simulink model "untitled"  (R2024b)
settings: Solver=FixedStepAuto  StartTime=0.0  StopTime=100  FixedStep=0.001  RelTol=1e-3  EnableMultiTasking=on
libraries: arduinolib x4
settings Model: ExtModeTrigDuration=2  Creator=abdal  LastModifiedBy=abdal
settings SolverCC: AutoInsertRateTranBlk=on
settings OptimizationCC: EnhancedBackFolding=on  PassReuseOutputArgsAs=Individual arguments  ZeroExternalMemoryAtStartup=off  ZeroInternalMemoryAtStartup=off  MaxStackSize=64  OptimizeBlockOrder=speed  DifferentSizesBufferReuse=on  OptimizationCustomize=off  EfficientTunableParamExpr=on
settings DebuggingCC: ParameterTunabilityLossMsg=error
settings HardwareCC: ProdBitPerInt=16  ProdBitPerPointer=16  ProdBitPerSizeT=16  ProdBitPerPtrDiffT=16  ProdLargestAtomicFloat=None  ProdWordSize=8  ProdHWDeviceType=Atmel->AVR
settings SFSimCC: MATLABDynamicMemAlloc=off
settings RTWCC: Description=Embedded Coder  SystemTargetFile=ert.tlc  HardwareBoard=Arduino Uno  TemplateMakefile=ert_default_tmf  Toolchain=Arduino AVR  BuildConfiguration=Faster Runs
settings CodeAppCC: ForceParamTrailComments=on  IgnoreCustomStorageClasses=off  OperatorAnnotations=on  SimulinkDataObjDesc=on  SFDataObjDesc=on  InsertBlockDesc=on
settings ERTTargetCC: SupportContinuousTime=on  SupportVariableSizeSignals=on  ExtModeTransport=3  ExtModeStaticAlloc=on  ExtModeAutomaticAllocSize=off  ExtModeStaticAllocSize=250  ExtModeMexFile=ext_xcp  ExtModeIntrfLevel=Level2 - Open  InlinedParameterPlacement=Hierarchical

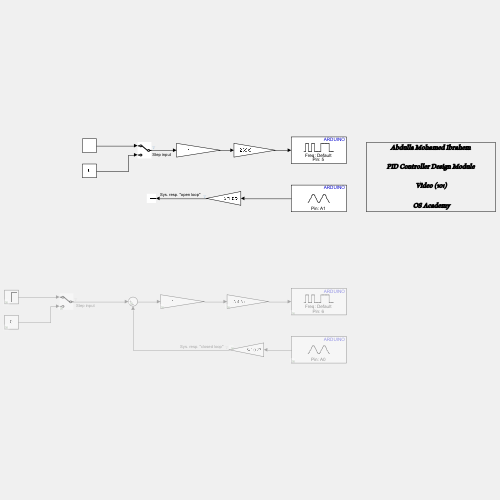
[thumbnail: Simulink's stored preview of the top-level diagram]
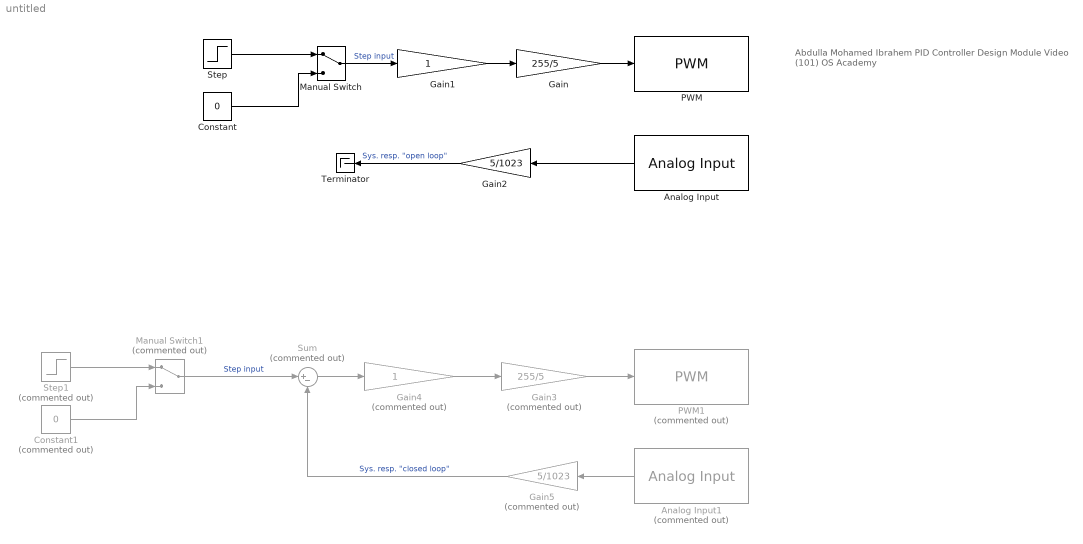
== system untitled ==
  note: Abdulla Mohamed Ibrahem
      | PID Controller Design Module
      | Video (101)
      | OS Academy
  Analog Input : arduinolib/Analog Input  pinNumber=1  ReadResultsOnly=off  ConversionTriggerSource=Software  ExternalTriggerType=uint32( 0 )  OutputDataType=uint16  EnableConversionCompleteNotify=off  EnableOuputStatus=off  SampleTime=-1  blockPlatform=arduino
  Analog Input1 : arduinolib/Analog Input  Commented=on  pinNumber=0  ReadResultsOnly=off  ConversionTriggerSource=Software  ExternalTriggerType=uint32( 0 )  OutputDataType=uint16  EnableConversionCompleteNotify=off  EnableOuputStatus=off  SampleTime=-1  blockPlatform=arduino
  Constant : Constant  Value=0
  Constant1 : Constant  Commented=on  Value=0
  Gain : Gain  Gain=255/5
  Gain1 : Gain
  Gain2 : Gain  Gain=5/1023
  Gain3 : Gain  Commented=on  Gain=255/5
  Gain4 : Gain  Commented=on
  Gain5 : Gain  Commented=on  Gain=5/1023
  Manual Switch : ManualSwitch
  Manual Switch1 : ManualSwitch  Commented=on
  PWM : arduinolib/PWM  pinNumber=5  frequencyType=Default  desiredFrequency=490.2  achievableFrequency=490.2
  PWM1 : arduinolib/PWM  Commented=on  pinNumber=6  frequencyType=Default  desiredFrequency=490.2  achievableFrequency=490.2
  Step : Step  Time=0.5  SampleTime=0
  Step1 : Step  Commented=on  Time=2  SampleTime=0
  Sum : Sum  Commented=on  Inputs=|+-
  Terminator : Terminator
  wires:
  Gain/1 -> PWM/1
  Gain1/1 -> Gain/1
  Analog Input/1 -> Gain2/1
  Constant/1 -> Manual Switch/2
  Step/1 -> Manual Switch/1
  Manual Switch/1 -> Gain1/1  "Step input"
  Gain2/1 -> Terminator/1  "Sys. resp. \"open loop\""
  Step1/1 -> Manual Switch1/1
  Constant1/1 -> Manual Switch1/2
  Analog Input1/1 -> Gain5/1
  Gain4/1 -> Gain3/1
  Gain3/1 -> PWM1/1
  Manual Switch1/1 -> Sum/1  "Step input"
  Sum/1 -> Gain4/1
  Gain5/1 -> Sum/2  "Sys. resp. \"closed loop\""
